simulink model "franka_placement_task"  (R2020b)
settings: Solver=FixedStepAuto  StartTime=0.0  StopTime=20  FixedStep=0.01  RelTol=1e-3
values from neighbouring files (symbols this model uses):
  a0 = 0.99    [init.m]
  berta = 0.98    [init.m]
  csi = 1    [init.m]
  e_max = 0.01    [init.m]
  F_int_max = 5    [init.m]
  F_max = 2    [init.m]
  g = 9.81    [init.m]
  k_can = 500    [init.m]
  k_shelf = k_table    (= 10000)    [init.m]
  k_table = 10000    [init.m]
  k_wall = k_table    (= 10000)    [init.m]
  l_can = 0.1    [init.m]
  M = 1    [init.m]
  mass = 1    [init.m]
  mass_can = 0.5    [init.m]
  q_max = q_max - deg2rad([0 0 0 10 0 5 0])    [init.m]
  q_min = q_min + deg2rad([0 0 0 10 0 5 0])    [init.m]
  y_can = 0.2    [init.m]
  y_wall = -0.3    [init.m]
  z_shelf = 0.3+0.043    (= 0.343)    [init.m]
  z_table = 0+0.043    (= 0.043)    [init.m]
(part 1 of 2)
settings Model: Creator=Rachele  LastModifiedBy=giorg

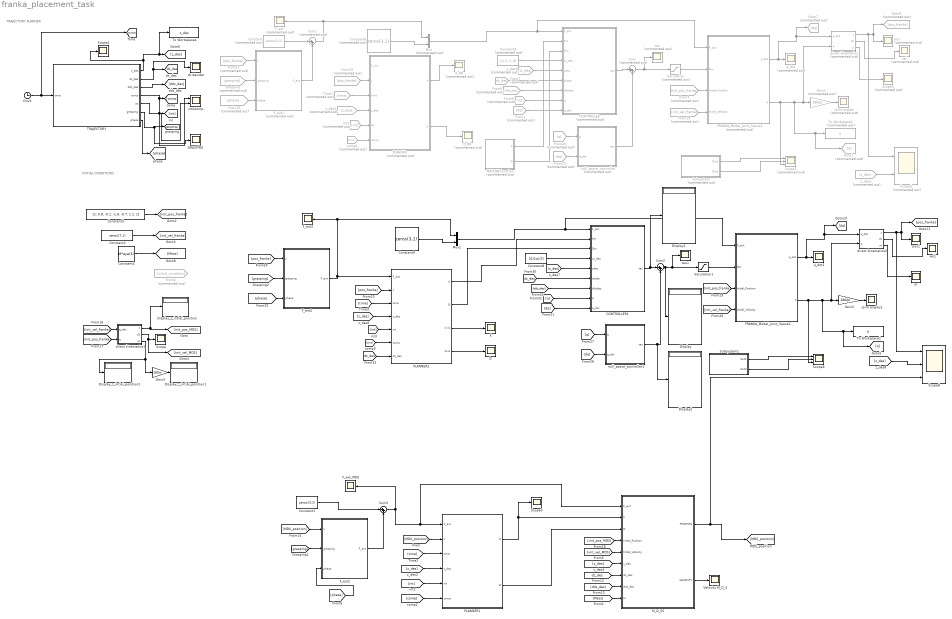
== system franka_placement_task ==
  note: TRAJECTORY PLANNER
  note: INITIAL CONDITIONS
  CONTROLLER : MATLAB Function  Commented=on  TreatAsAtomicUnit=on
  CONTROLLER1 : MATLAB Function  TreatAsAtomicUnit=on
  Clock : Clock
  Constant : Constant  Commented=on  Value=zeros(3,1)
  Constant1 : Constant  Value=zeros(3,1)
  Constant2 : Constant  Value=zeros(7,1)
  Constant3 : Constant  Value=[1; 0.8; -0.1; -1.6; -0.7; 1.1; 1]  VectorParams1D=off
  Constant4 : Constant  Value=M*eye(3)
  Constant5 : Constant  Commented=on  Value=[-2.3; 1; 0]
  Constant6 : Constant  Commented=on  Value=zeros(3,1)
  Constant8 : Constant  Value=[0;0;pi/2]
  Constant9 : Constant  Value=zeros(3,1)
  D : Scope
  D_RR : Scope  Commented=on
  Display : Display
  Display1 : Display
  Display2 : Display
  Display_z_intial_position : Display
  Display_z_intial_position1 : Display
  Display_z_intial_position2 : Display
  FRANKA_Model_Joint_Space1 : Subsystem  Commented=on
  FRANKA_Model_Joint_Space2 : Subsystem
  F_ext : Scope  Commented=on
  F_ext1 : MATLAB Function  Commented=on  TreatAsAtomicUnit=on
  F_ext2 : MATLAB Function  TreatAsAtomicUnit=on
  F_ext3 : Scope
  F_ext4 : MATLAB Function  TreatAsAtomicUnit=on
  F_ext_MDS : Scope
  From1 : From  Commented=on  GotoTag=dq
  From10 : From  Commented=on  GotoTag=pos_franka
  From11 : From  Commented=on  GotoTag=pos_franka
  From15 : From  Commented=on  GotoTag=phase
  From19 : From  Commented=on  GotoTag=init_vel_franka
  From20 : From  Commented=on  GotoTag=q
  From22 : From  Commented=on  GotoTag=dq
  From3 : From  Commented=on  GotoTag=init_pos_franka
  From4 : From  Commented=on  GotoTag=initial_condition
  From7 : From  Commented=on  GotoTag=dz_des  TagVisibility=global
  From8 : From  Commented=on  GotoTag=ddz_des
  From9 : From  Commented=on  GotoTag=q
  GRASPING : Scope
  Gain1 : Gain  Commented=on  Gain=180/pi
  Gain2 : Gain  Gain=180/pi
  Gain3 : Gain  Gain=180/pi
  Goto1 : Goto  Commented=on  GotoTag=q
  Goto7 : Goto  Commented=on  GotoTag=dq
  Goto9 : Goto  Commented=on  GotoTag=pos_franka
  Grasping : From  Commented=on  GotoTag=grasping
  Joint angles : Scope  Commented=on
  Joint angles1 : Scope
  K : Scope
  K_RR : Scope  Commented=on
  MATLAB Function : MATLAB Function  Commented=on  TreatAsAtomicUnit=on
  M_D_S5 : Subsystem
  Mux : Mux  Commented=on  Inputs=2
  Mux1 : Mux  Inputs=2
  PLANNER : Subsystem  Commented=on
  PLANNER1 : Subsystem
  PLANNER2 : Subsystem
  Saturation : Saturate  Commented=on  UpperLimit=100  LowerLimit=-100
  Saturation1 : Saturate  UpperLimit=100  LowerLimit=-100
  Scope : Scope
  Scope1 : Scope  Commented=on  NumInputPorts=3
  Scope2 : Scope  Commented=on
  Scope3 : Scope
  Scope4 : Scope
  Scope5 : Scope  Commented=on  NumInputPorts=2
  Scope6 : Scope  NumInputPorts=3
  Scope8 : Scope  NumInputPorts=3
  Subsystem : Subsystem  Commented=on
  Subsystem1 : Subsystem
  Sum : Sum  Commented=on  Inputs=|++
  Sum1 : Sum  Commented=on  Inputs=|++
  Sum2 : Sum  Inputs=|++
  Sum3 : Sum  Inputs=|++
  TRAJECTORY : Subsystem
  Time1 : From  Commented=on  GotoTag=time
  To Workspace1 : ToWorkspace  VariableName=q  SaveFormat=Timeseries  SampleTime=-1
  To Workspace2 : ToWorkspace  Commented=on  VariableName=q  SaveFormat=Timeseries  SampleTime=-1
  To Workspace4 : ToWorkspace  VariableName=z_des  SaveFormat=Timeseries  SampleTime=-1
      settings: Save2DSignal=2-D array (concatenate along first dimension)
  Velocity M_D_S : Scope
  comp1 : From  Commented=on  GotoTag=comp
  direct kinematics : MATLAB Function  Commented=on  TreatAsAtomicUnit=on
  direct kinematics1 : MATLAB Function  TreatAsAtomicUnit=on
  direct kinematics2 : MATLAB Function  TreatAsAtomicUnit=on
  dz desider : Scope
  int&comp : Scope  NumInputPorts=2
  int1 : From  Commented=on  GotoTag=int
  null_space_controller : MATLAB Function  Commented=on  TreatAsAtomicUnit=on
  null_space_controller1 : MATLAB Function  TreatAsAtomicUnit=on
  or : Scope
  pos : Scope  Commented=on
  pos1 : Scope
  q_dot : Scope  Commented=on
  q_dot1 : Scope
  tau : Scope  Commented=on
  tau1 : Scope
  vel : Scope  Commented=on
  vel1 : Scope
  z_des1 : From  Commented=on  GotoTag=z_des
  z_des3 : From  Commented=on  GotoTag=z_des
  z_des5 : From  Commented=on  GotoTag=z_des
  tag scope: dz_des=global
  wires:
  TRAJECTORY/1(z_des) -> [z_des], To Workspace4/1, Scope4/1
  Sum3/1 -> F_ext_MDS/1, M_D_S5/1(F_ext), PLANNER1/1(F_ext)
  null_space_controller/1(tau) -> Sum/2
  Sum1/1 -> Mux/1, F_ext/1
  Subsystem/2(Out2) -> Scope1/2
  comp1/1 -> PLANNER/6(comp)
  [int] -> PLANNER1/5(int)
  F_ext2/1(F_ext) -> Sum3/2
  PLANNER/1(K) -> K_RR/1
  F_ext1/1(F_ext) -> Sum1/2
  Subsystem/1(Out1) -> Scope1/1
  PLANNER1/1(K) -> M_D_S5/2(K), Scope3/1
  [init_vel_franka] -> direct kinematics1/1(q_dot)
  From11/1 -> F_ext1/1(z)
  Gain1/1 -> Joint angles/1
  Constant1/1 -> Sum3/1
  Constant3/1 -> [init_pos_franka]
  From8/1 -> CONTROLLER/7(ddzdes)
  [phase] -> F_ext2/3(phase)
  Constant/1 -> Sum1/1
  [MDS_position] -> PLANNER1/2(z)
  Saturation/1 -> FRANKA_Model_Joint_Space1/2(tau)
  Grasping/1 -> F_ext1/2(grasping)
  Clock/1 -> TRAJECTORY/1(time), [time]
  [init_vel_MDS] -> M_D_S5/5(Initial_Velocity)
  From20/1 -> null_space_controller/1(q)
  CONTROLLER/1(tau) -> Sum/1
  PLANNER/2(D) -> D_RR/1
  z_des3/1 -> CONTROLLER/5(zdes)
  FRANKA_Model_Joint_Space1/2(q) -> Scope1/3, Goto1/1, To Workspace2/1, direct kinematics/2(q), Gain1/1
  Sum/1 -> Saturation/1, tau/1
  From3/1 -> FRANKA_Model_Joint_Space1/3(Initial_Position)
  direct kinematics1/1(z) -> [init_pos_MDS], Display_z_intial_position/1
  Constant4/1 -> [Mass]
  TRAJECTORY/5(int) -> int&comp/2, [int]
  [init_pos_franka] -> direct kinematics1/2(q)
  direct kinematics/1(z) -> Scope5/1, pos/1, Goto9/1
  From19/1 -> FRANKA_Model_Joint_Space1/4(Initial_Velocity)
  FRANKA_Model_Joint_Space1/1(q_dot) -> Goto7/1, direct kinematics/1(q_dot), q_dot/1
  [dz_des] -> M_D_S5/7(dz_des)
  int1/1 -> PLANNER/5(int)
  [z_des] -> PLANNER1/4(z_des)
  [comp] -> PLANNER1/6(comp)
  [ddz_des] -> M_D_S5/8(ddz_des)
  Time1/1 -> PLANNER/3(time)
  M_D_S5/2(VELOCITY) -> Velocity M_D_S/1
  TRAJECTORY/4(comp) -> int&comp/1, [comp]
  z_des1/1 -> PLANNER/4(z_des)
  From15/1 -> F_ext1/3(phase)
  [time] -> PLANNER1/3(time)
  TRAJECTORY/3(ddz_des) -> [ddz_des]
  [Mass] -> M_D_S5/9(M)
  TRAJECTORY/7(phase) -> [phase]
  [init_pos_MDS] -> M_D_S5/4(Initial_Position)
  TRAJECTORY/2(dz_des) -> dz desider/1, [dz_des]
  direct kinematics/2(dz) -> vel/1
  [MDS_position] -> F_ext2/1(z)
  Constant2/1 -> [init_vel_franka]
  From10/1 -> PLANNER/2(z)
  From9/1 -> CONTROLLER/8(q)
  [z_des] -> M_D_S5/6(z_des)
  TRAJECTORY/6(grasping) -> GRASPING/1, [grasping]
  M_D_S5/1(POSITION) -> Scope8/3, [MDS_position]
  From7/1 -> CONTROLLER/6(dzdes)
  From1/1 -> CONTROLLER/9(q_dot)
  From22/1 -> null_space_controller/2(q_dot)
  [grasping] -> F_ext2/2(grasping)
  Constant5/1 -> CONTROLLER/4(or_des)
  MATLAB Function/1(K) -> CONTROLLER/2(Km)
  MATLAB Function/2(D) -> CONTROLLER/3(Dm)
  direct kinematics/3(or) -> Scope2/1
  z_des5/1 -> Scope5/2
  Constant6/1 -> Mux/2
  Mux/1 -> FRANKA_Model_Joint_Space1/1(F_ext), CONTROLLER/1(F_ext)
  [comp] -> PLANNER2/6(comp)
  Subsystem1/1(Out1) -> Scope6/1
  Mux1/1 -> FRANKA_Model_Joint_Space2/1(F_ext), CONTROLLER1/1(F_ext)
  Constant9/1 -> Mux1/2
  direct kinematics2/3(or) -> or/1
  Constant8/1 -> CONTROLLER1/4(or_des)
  [dq] -> CONTROLLER1/9(q_dot)
  direct kinematics2/2(dz) -> vel1/1
  [ddz_des] -> CONTROLLER1/7(ddzdes)
  [z_des] -> PLANNER2/4(z_des)
  Gain2/1 -> Joint angles1/1
  [dq] -> null_space_controller1/2(q_dot)
  [pos_franka] -> F_ext4/1(z)
  [phase] -> F_ext4/3(phase)
  [time] -> PLANNER2/3(time)
  [pos_franka] -> PLANNER2/2(z)
  [init_pos_franka] -> FRANKA_Model_Joint_Space2/3(Initial_Position)
  FRANKA_Model_Joint_Space2/1(q_dot) -> [dq], direct kinematics2/1(q_dot), q_dot1/1
  direct kinematics2/1(z) -> Scope8/1, pos1/1, [pos_franka]
  [int] -> PLANNER2/5(int)
  [z_des] -> Scope8/2
  [z_des] -> CONTROLLER1/5(zdes)
  null_space_controller1/1(tau) -> Display2/1, Sum2/2
  [grasping] -> F_ext4/2(grasping)
  Sum2/1 -> Display/1, Saturation1/1, tau1/1
  PLANNER2/1(K) -> CONTROLLER1/2(Km)
  FRANKA_Model_Joint_Space2/2(q) -> Scope6/3, [q], To Workspace1/1, direct kinematics2/2(q), Gain2/1
  [dz_des] -> CONTROLLER1/6(dzdes)
  [q] -> null_space_controller1/1(q)
  PLANNER2/2(D) -> CONTROLLER1/3(Dm)
  [init_vel_franka] -> FRANKA_Model_Joint_Space2/4(Initial_Velocity)
  CONTROLLER1/1(tau) -> Display1/1, Sum2/1
  Saturation1/1 -> FRANKA_Model_Joint_Space2/2(tau)
  Subsystem1/2(Out2) -> Scope6/2
  [q] -> CONTROLLER1/8(q)
  PLANNER1/2(D) -> M_D_S5/3(D)
  direct kinematics1/2(dz) -> Scope/1, [init_vel_MDS]
  Gain3/1 -> Display_z_intial_position1/1
  direct kinematics1/3(or) -> Display_z_intial_position2/1, Gain3/1
  F_ext4/1(F_ext) -> PLANNER2/1(F_ext), F_ext3/1, Mux1/1
  PLANNER2/3(kvis) -> K/1
  PLANNER2/4(dvis) -> D/1
  [dz_des] -> PLANNER2/7(dz_des)

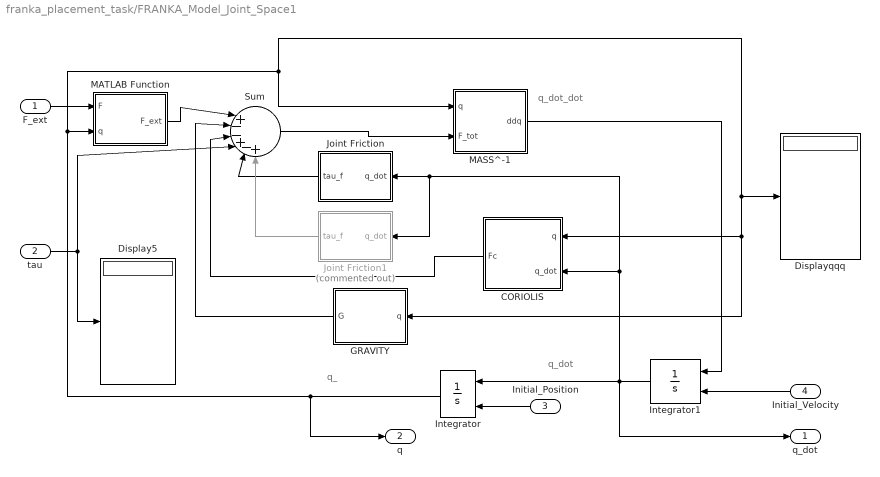
== system franka_placement_task/FRANKA_Model_Joint_Space1 ==
  note: q_dot
  note: q_dot_dot
  note: q_
  F_ext : Inport
  tau : Inport  Port=2
  Initial_Position : Inport  Port=3
  Initial_Velocity : Inport  Port=4
  CORIOLIS : MATLAB Function  TreatAsAtomicUnit=on
  Display5 : Display
  Displayqqq : Display
  GRAVITY : MATLAB Function  TreatAsAtomicUnit=on
  Integrator : Integrator  InitialConditionSource=external
  Integrator1 : Integrator  InitialConditionSource=external  InitialCondition=[0;0]
  Joint Friction : MATLAB Function  TreatAsAtomicUnit=on
  Joint Friction1 : MATLAB Function  Commented=on  TreatAsAtomicUnit=on
  MASS^-1 : MATLAB Function  TreatAsAtomicUnit=on
  MATLAB Function : MATLAB Function  TreatAsAtomicUnit=on
  Sum : Sum  Inputs=||+--+-+
  q_dot : Outport
  q : Outport  Port=2
  wires:
  GRAVITY/1(G) -> Sum/2
  MATLAB Function/1(F_ext) -> Sum/1
  Initial_Position/1 -> Integrator/2
  F_ext/1 -> MATLAB Function/1(F)
  Integrator/1 -> MASS^-1/1(q), GRAVITY/1(q), CORIOLIS/1(q), Displayqqq/1, MATLAB Function/2(q), q/1
  Integrator1/1 -> q_dot/1, CORIOLIS/2(q_dot), Joint Friction1/1(q_dot), Joint Friction/1(q_dot), Integrator/1
  Initial_Velocity/1 -> Integrator1/2
  MASS^-1/1(ddq) -> Integrator1/1
  Sum/1 -> MASS^-1/2(F_tot)
  CORIOLIS/1(Fc) -> Sum/3
  tau/1 -> Display5/1, Sum/4
  Joint Friction/1(tau_f) -> Sum/5
  Joint Friction1/1(tau_f) -> Sum/6

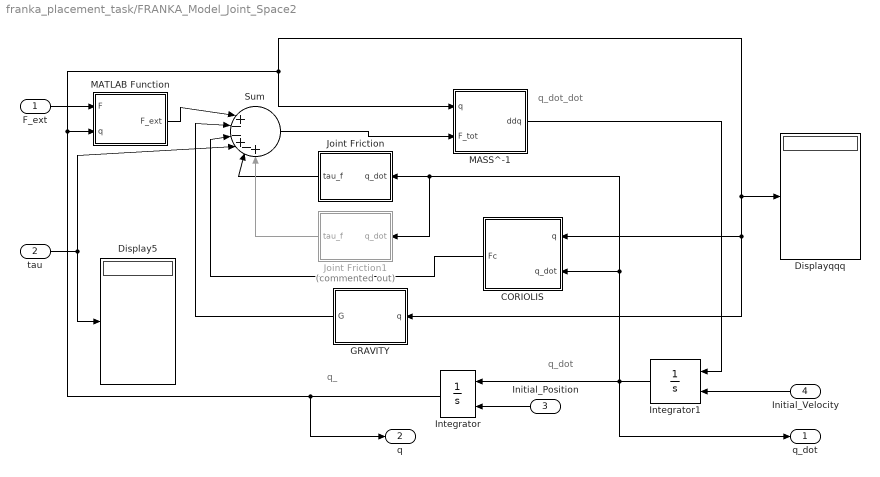
== system franka_placement_task/FRANKA_Model_Joint_Space2 ==
  note: q_dot
  note: q_dot_dot
  note: q_
  F_ext : Inport
  tau : Inport  Port=2
  Initial_Position : Inport  Port=3
  Initial_Velocity : Inport  Port=4
  CORIOLIS : MATLAB Function  TreatAsAtomicUnit=on
  Display5 : Display
  Displayqqq : Display
  GRAVITY : MATLAB Function  TreatAsAtomicUnit=on
  Integrator : Integrator  InitialConditionSource=external
  Integrator1 : Integrator  InitialConditionSource=external  InitialCondition=[0;0]
  Joint Friction : MATLAB Function  TreatAsAtomicUnit=on
  Joint Friction1 : MATLAB Function  Commented=on  TreatAsAtomicUnit=on
  MASS^-1 : MATLAB Function  TreatAsAtomicUnit=on
  MATLAB Function : MATLAB Function  TreatAsAtomicUnit=on
  Sum : Sum  Inputs=||+--+-+
  q_dot : Outport
  q : Outport  Port=2
  wires:
  GRAVITY/1(G) -> Sum/2
  MATLAB Function/1(F_ext) -> Sum/1
  Initial_Position/1 -> Integrator/2
  F_ext/1 -> MATLAB Function/1(F)
  Integrator/1 -> MASS^-1/1(q), GRAVITY/1(q), CORIOLIS/1(q), Displayqqq/1, MATLAB Function/2(q), q/1
  Integrator1/1 -> q_dot/1, CORIOLIS/2(q_dot), Joint Friction1/1(q_dot), Joint Friction/1(q_dot), Integrator/1
  Initial_Velocity/1 -> Integrator1/2
  MASS^-1/1(ddq) -> Integrator1/1
  Sum/1 -> MASS^-1/2(F_tot)
  CORIOLIS/1(Fc) -> Sum/3
  tau/1 -> Display5/1, Sum/4
  Joint Friction/1(tau_f) -> Sum/5
  Joint Friction1/1(tau_f) -> Sum/6

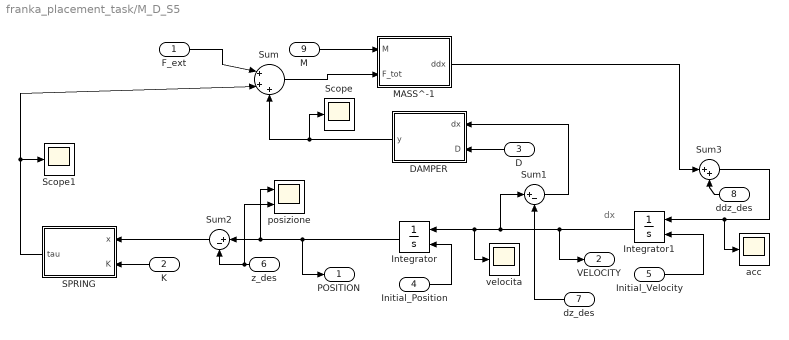
== system franka_placement_task/M_D_S5 ==
  note: dx
  F_ext : Inport
  K : Inport  Port=2
  D : Inport  Port=3
  Initial_Position : Inport  Port=4
  Initial_Velocity : Inport  Port=5
  z_des : Inport  Port=6
  dz_des : Inport  Port=7
  ddz_des : Inport  Port=8
  M : Inport  Port=9
  DAMPER : MATLAB Function  TreatAsAtomicUnit=on
  Integrator : Integrator  InitialConditionSource=external
  Integrator1 : Integrator  InitialConditionSource=external
  MASS^-1 : MATLAB Function  TreatAsAtomicUnit=on
  SPRING : MATLAB Function  TreatAsAtomicUnit=on
  Scope : Scope
  Scope1 : Scope
  Sum : Sum  Inputs=|+++
  Sum1 : Sum  Inputs=|+-
  Sum2 : Sum  Inputs=|+-
  Sum3 : Sum  Inputs=|++
  acc : Scope
  posizione : Scope  NumInputPorts=2
  velocita : Scope
  POSITION : Outport
  VELOCITY : Outport  Port=2
  wires:
  Integrator1/1 -> velocita/1, Integrator/1, Sum1/1, VELOCITY/1
  SPRING/1(tau) -> Sum/2, Scope1/1
  Integrator/1 -> posizione/1, Sum2/1, POSITION/1
  DAMPER/1(y) -> Scope/1, Sum/3
  Sum/1 -> MASS^-1/2(F_tot)
  M/1 -> MASS^-1/1(M)
  D/1 -> DAMPER/2(D)
  K/1 -> SPRING/2(K)
  Initial_Velocity/1 -> Integrator1/2
  Initial_Position/1 -> Integrator/2
  z_des/1 -> posizione/2, Sum2/2
  Sum2/1 -> SPRING/1(x)
  MASS^-1/1(ddx) -> Sum3/1
  Sum1/1 -> DAMPER/1(dx)
  Sum3/1 -> acc/1, Integrator1/1
  dz_des/1 -> Sum1/2
  ddz_des/1 -> Sum3/2
  F_ext/1 -> Sum/1

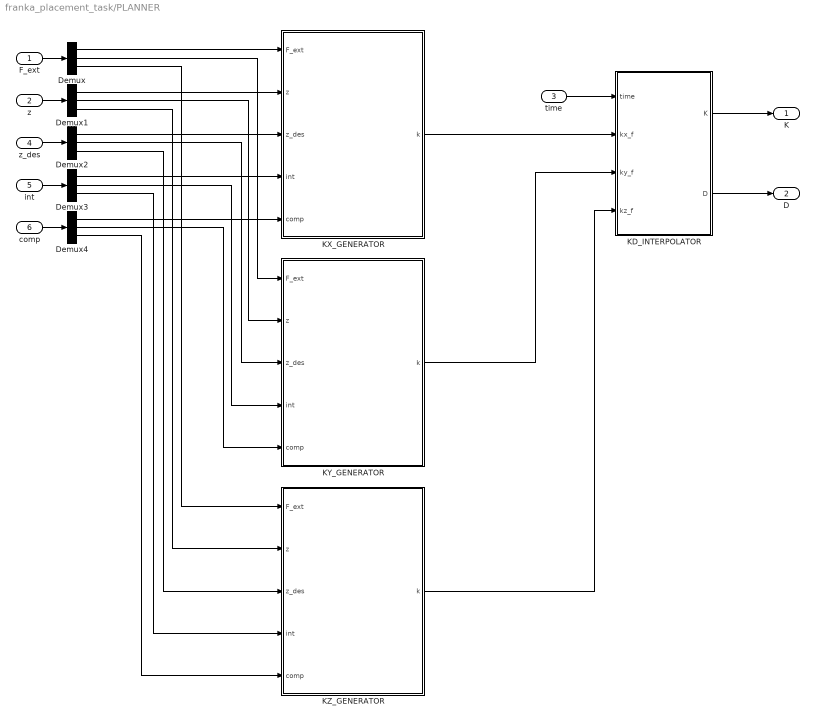
== system franka_placement_task/PLANNER ==
  F_ext : Inport
  z : Inport  Port=2
  time : Inport  Port=3
  z_des : Inport  Port=4
  int : Inport  Port=5
  comp : Inport  Port=6
  Demux{,1..4} (5 alike) : Demux  Outputs=3
  "KD_INTERPOLATOR " : MATLAB Function  TreatAsAtomicUnit=on
  KX_GENERATOR : MATLAB Function  TreatAsAtomicUnit=on
  KY_GENERATOR : MATLAB Function  TreatAsAtomicUnit=on
  KZ_GENERATOR : MATLAB Function  TreatAsAtomicUnit=on
  K : Outport
  D : Outport  Port=2
  wires:
  time/1 -> "KD_INTERPOLATOR "/1(time)
  "KD_INTERPOLATOR "/2(D) -> D/1
  "KD_INTERPOLATOR "/1(K) -> K/1
  KX_GENERATOR/1(k) -> "KD_INTERPOLATOR "/2(kx_f)
  Demux/1 -> KX_GENERATOR/1(F_ext)
  Demux1/1 -> KX_GENERATOR/2(z)
  Demux2/1 -> KX_GENERATOR/3(z_des)
  Demux3/1 -> KX_GENERATOR/4(int)
  Demux4/1 -> KX_GENERATOR/5(comp)
  F_ext/1 -> Demux/1
  z/1 -> Demux1/1
  z_des/1 -> Demux2/1
  int/1 -> Demux3/1
  comp/1 -> Demux4/1
  Demux/2 -> KY_GENERATOR/1(F_ext)
  Demux1/2 -> KY_GENERATOR/2(z)
  Demux2/2 -> KY_GENERATOR/3(z_des)
  Demux3/2 -> KY_GENERATOR/4(int)
  Demux4/2 -> KY_GENERATOR/5(comp)
  Demux/3 -> KZ_GENERATOR/1(F_ext)
  Demux1/3 -> KZ_GENERATOR/2(z)
  Demux2/3 -> KZ_GENERATOR/3(z_des)
  Demux3/3 -> KZ_GENERATOR/4(int)
  Demux4/3 -> KZ_GENERATOR/5(comp)
  KY_GENERATOR/1(k) -> "KD_INTERPOLATOR "/3(ky_f)
  KZ_GENERATOR/1(k) -> "KD_INTERPOLATOR "/4(kz_f)

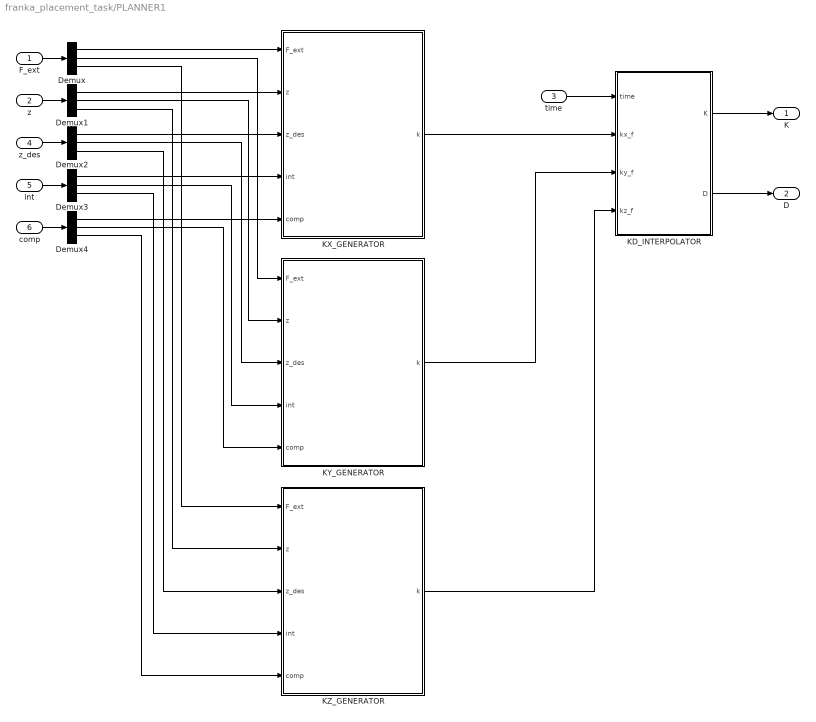
== system franka_placement_task/PLANNER1 ==
  F_ext : Inport
  z : Inport  Port=2
  time : Inport  Port=3
  z_des : Inport  Port=4
  int : Inport  Port=5
  comp : Inport  Port=6
  Demux{,1..4} (5 alike) : Demux  Outputs=3
  "KD_INTERPOLATOR " : MATLAB Function  TreatAsAtomicUnit=on
  KX_GENERATOR : MATLAB Function  TreatAsAtomicUnit=on
  KY_GENERATOR : MATLAB Function  TreatAsAtomicUnit=on
  KZ_GENERATOR : MATLAB Function  TreatAsAtomicUnit=on
  K : Outport
  D : Outport  Port=2
  wires:
  KZ_GENERATOR/1(k) -> "KD_INTERPOLATOR "/4(kz_f)
  KY_GENERATOR/1(k) -> "KD_INTERPOLATOR "/3(ky_f)
  Demux4/3 -> KZ_GENERATOR/5(comp)
  Demux3/3 -> KZ_GENERATOR/4(int)
  Demux2/3 -> KZ_GENERATOR/3(z_des)
  Demux1/3 -> KZ_GENERATOR/2(z)
  Demux/3 -> KZ_GENERATOR/1(F_ext)
  Demux4/2 -> KY_GENERATOR/5(comp)
  Demux3/2 -> KY_GENERATOR/4(int)
  Demux2/2 -> KY_GENERATOR/3(z_des)
  Demux1/2 -> KY_GENERATOR/2(z)
  Demux/2 -> KY_GENERATOR/1(F_ext)
  comp/1 -> Demux4/1
  int/1 -> Demux3/1
  z_des/1 -> Demux2/1
  z/1 -> Demux1/1
  F_ext/1 -> Demux/1
  Demux4/1 -> KX_GENERATOR/5(comp)
  Demux3/1 -> KX_GENERATOR/4(int)
  Demux2/1 -> KX_GENERATOR/3(z_des)
  Demux1/1 -> KX_GENERATOR/2(z)
  Demux/1 -> KX_GENERATOR/1(F_ext)
  KX_GENERATOR/1(k) -> "KD_INTERPOLATOR "/2(kx_f)
  "KD_INTERPOLATOR "/1(K) -> K/1
  "KD_INTERPOLATOR "/2(D) -> D/1
  time/1 -> "KD_INTERPOLATOR "/1(time)

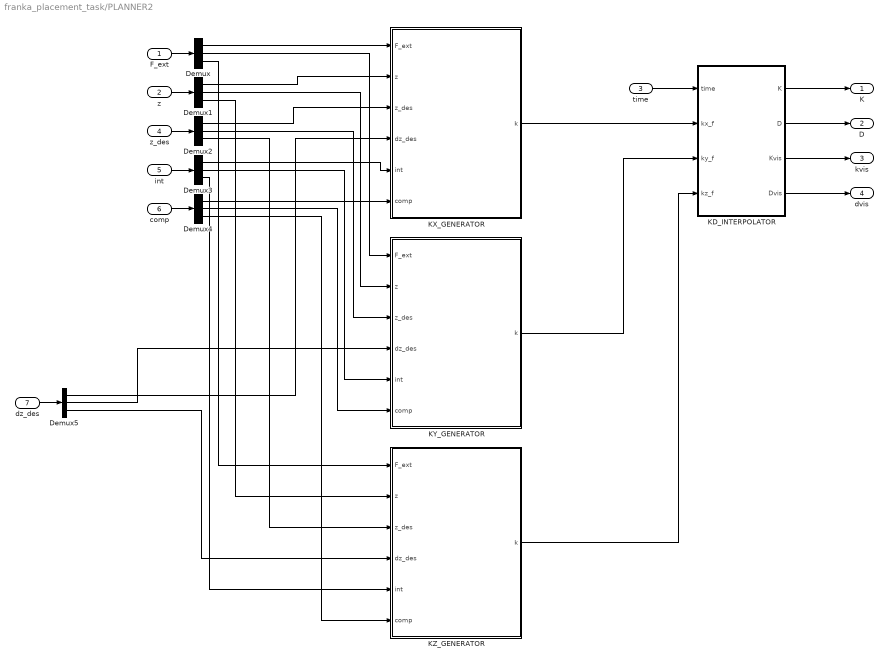
== system franka_placement_task/PLANNER2 ==
  F_ext : Inport
  z : Inport  Port=2
  time : Inport  Port=3
  z_des : Inport  Port=4
  int : Inport  Port=5
  comp : Inport  Port=6
  dz_des : Inport  Port=7
  Demux{,1..5} (6 alike) : Demux  Outputs=3
  "KD_INTERPOLATOR " : MATLAB Function  TreatAsAtomicUnit=on
  KX_GENERATOR : MATLAB Function  TreatAsAtomicUnit=on
  KY_GENERATOR : MATLAB Function  TreatAsAtomicUnit=on
  KZ_GENERATOR : MATLAB Function  TreatAsAtomicUnit=on
  K : Outport
  D : Outport  Port=2
  kvis : Outport  Port=3
  dvis : Outport  Port=4
  wires:
  time/1 -> "KD_INTERPOLATOR "/1(time)
  "KD_INTERPOLATOR "/2(D) -> D/1
  "KD_INTERPOLATOR "/1(K) -> K/1
  KX_GENERATOR/1(k) -> "KD_INTERPOLATOR "/2(kx_f)
  Demux/1 -> KX_GENERATOR/1(F_ext)
  Demux1/1 -> KX_GENERATOR/2(z)
  Demux2/1 -> KX_GENERATOR/3(z_des)
  Demux3/1 -> KX_GENERATOR/5(int)
  Demux4/1 -> KX_GENERATOR/6(comp)
  F_ext/1 -> Demux/1
  z/1 -> Demux1/1
  z_des/1 -> Demux2/1
  int/1 -> Demux3/1
  comp/1 -> Demux4/1
  Demux/2 -> KY_GENERATOR/1(F_ext)
  Demux1/2 -> KY_GENERATOR/2(z)
  Demux2/2 -> KY_GENERATOR/3(z_des)
  Demux3/2 -> KY_GENERATOR/5(int)
  Demux4/2 -> KY_GENERATOR/6(comp)
  Demux/3 -> KZ_GENERATOR/1(F_ext)
  Demux1/3 -> KZ_GENERATOR/2(z)
  Demux2/3 -> KZ_GENERATOR/3(z_des)
  Demux3/3 -> KZ_GENERATOR/5(int)
  Demux4/3 -> KZ_GENERATOR/6(comp)
  KY_GENERATOR/1(k) -> "KD_INTERPOLATOR "/3(ky_f)
  KZ_GENERATOR/1(k) -> "KD_INTERPOLATOR "/4(kz_f)
  "KD_INTERPOLATOR "/3(Kvis) -> kvis/1
  "KD_INTERPOLATOR "/4(Dvis) -> dvis/1
  dz_des/1 -> Demux5/1
  Demux5/3 -> KZ_GENERATOR/4(dz_des)
  Demux5/1 -> KX_GENERATOR/4(dz_des)
  Demux5/2 -> KY_GENERATOR/4(dz_des)

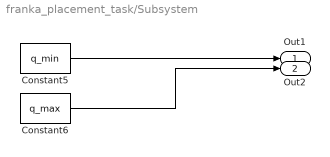
== system franka_placement_task/Subsystem ==
  Constant5 : Constant  Value=q_min
  Constant6 : Constant  Value=q_max
  Out1 : Outport
  Out2 : Outport  Port=2
  wires:
  Constant5/1 -> Out1/1
  Constant6/1 -> Out2/1

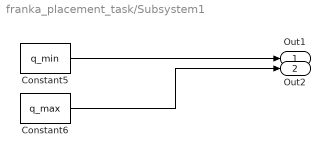
== system franka_placement_task/Subsystem1 ==
  Constant5 : Constant  Value=q_min
  Constant6 : Constant  Value=q_max
  Out1 : Outport
  Out2 : Outport  Port=2
  wires:
  Constant5/1 -> Out1/1
  Constant6/1 -> Out2/1

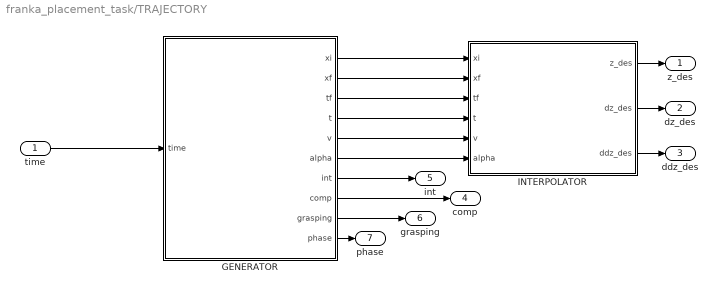
== system franka_placement_task/TRAJECTORY ==
  time : Inport
  GENERATOR : MATLAB Function  TreatAsAtomicUnit=on
  INTERPOLATOR : MATLAB Function  TreatAsAtomicUnit=on
  z_des : Outport
  dz_des : Outport  Port=2
  ddz_des : Outport  Port=3
  comp : Outport  Port=4
  int : Outport  Port=5
  grasping : Outport  Port=6
  phase : Outport  Port=7
  wires:
  GENERATOR/1(xi) -> INTERPOLATOR/1(xi)
  GENERATOR/2(xf) -> INTERPOLATOR/2(xf)
  GENERATOR/3(tf) -> INTERPOLATOR/3(tf)
  GENERATOR/4(t) -> INTERPOLATOR/4(t)
  GENERATOR/5(v) -> INTERPOLATOR/5(v)
  GENERATOR/6(alpha) -> INTERPOLATOR/6(alpha)
  INTERPOLATOR/1(z_des) -> z_des/1
  INTERPOLATOR/2(dz_des) -> dz_des/1
  INTERPOLATOR/3(ddz_des) -> ddz_des/1
  GENERATOR/7(int) -> int/1
  GENERATOR/8(comp) -> comp/1
  GENERATOR/9(grasping) -> grasping/1
  GENERATOR/10(phase) -> phase/1
  time/1 -> GENERATOR/1(time)

== matlab function franka_placement_task/PLANNER1/KD_INTERPOLATOR  ==
  settings: updateMethod=DISCRETE  sampleTime=Ts
  data: time input; K output; kx_f input; ky_f input; kz_f input; D output; e_max parameter; F_max parameter; M parameter; berta parameter; a0 parameter; mass parameter; csi parameter
function [K,D] = fcn(time, kx_f, ky_f, kz_f, e_max, F_max, M, berta, a0, mass, csi)
%% Description
% Interpolate K in order to guarantee stability

%% Outputs
% K             Stiffness matrix
% D             Damping matrix

%% Inputs
% kx_f, ky, f   desired values of K

%% Parameters
% F_max         nominal disturbance forces
% e_max         maximum steady-state error
% M             virtual mass
% berta, a0     parameters for the computation of stability conditions
% mass          virtual mass

%% persistent initialization
persistent kx ky kz time_prec
if isempty(time_prec)
    time_prec = 0;              % previous simulation time
end
if isempty(kx)
   kx = F_max/e_max;         % last value of k
end
if isempty(ky)
   ky = F_max/e_max;
end
if isempty(kz)
   kz = F_max/e_max;
end

% set k from desired one 
if kx_f <= kx       
    kx = kx_f;
else 
    % increese k in accordance with the stability conditions
    kx_i = kx;
    k_dotx = berta*(4*a0*sqrt(kx_i/mass)*(kx_i)^(3/2))/(sqrt(kx_i) + 2*a0*csi*sqrt(kx_i));
    k_tempx = kx_i + k_dotx*(time -time_prec);
    if k_tempx > kx_f
        kx = kx_f;
    else
        kx = k_tempx;
    end
end

% Y axes, same as X axes
if ky_f <= ky
    ky = ky_f;
else 
    ky_i = ky;
    k_doty = berta*(4*a0*sqrt(ky_i/mass)*(ky_i)^(3/2))/(sqrt(ky_i) + 2*a0*csi*sqrt(ky_i));
    k_tempy = ky_i + k_doty*(time -time_prec);
    if k_tempy > ky_f
        ky = ky_f;
    else
        ky = k_tempy;
    end
end

% Z axes, same as other axes
if kz_f <= kz
    kz = kz_f;
else 
    kz_i = kz;
    k_dotz = berta*(4*a0*sqrt(kz_i/mass)*(kz_i)^(3/2))/(sqrt(kz_i) + 2*a0*csi*sqrt(kz_i));
    k_tempz = kz_i + k_dotz*(time -time_prec);
    if k_tempz > kz_f
        kz = kz_f;
    else
        kz = k_tempz;
    end
end

time_prec = time;

% damping computation, critically damped condition
dx = sqrt(4*kx*M);
dy = sqrt(4*ky*M);
dz = sqrt(4*kz*M);

%% Final impedance matrices
D = diag([dx, dy, dz]);
K = diag([kx, ky, kz]);

end

== matlab function franka_placement_task/PLANNER1/KX_GENERATOR ==
  settings: updateMethod=DISCRETE  sampleTime=Ts
  data: k output; F_ext input; z input; z_des input; int input; comp input; e_max parameter; F_max parameter; F_int_max parameter
function k = fcn(F_ext, z, z_des, int, comp, e_max, F_max, F_int_max)
%% Description
% Set the K coefficient for a variable impedance controller based on a
% desired trajectory

%% Outputs
% k             stiffness

%% Inputs
% F_ext         measured external force
% z_des         desired trajectory
% z             current position
% int, comp     booleans for the interaction and compensation phase

%% Parameters
% F_int_max     desired interaction force
% F_max         nominal disturbance forces
% e_max         maximum steady-state error

%% persistent initialization
persistent ki kc F_comp int_prec comp_prec z_int z_int_dir 
if isempty(ki)
   ki = F_max/e_max;        % k obtained from interaction
end
if isempty(F_comp)
   F_comp = 0;              % weight to compensate
end
if isempty(kc)
      kc = F_max/e_max;     % k obtained from compensation
end
if isempty(z_int) 
    z_int = 1000;       % obstacle(or interaction) position
end
if isempty(z_int_dir) 
    z_int_dir = 0;          % prohibited direction due to the obstacle
end
if isempty(int_prec)
    int_prec = 0;           % previous values of int
end
if isempty(comp_prec)
    comp_prec = 0;          % previous values od comp
end

%% INTERACTION
% set ki in order to match a desired interaction force with the
% envirorment, and store interaction's position when detected
% X axes
if int == 1
    % detection of an interaction 
    if abs(F_ext-F_comp) > F_max
        if z_int == 1000                     % z_int has not been set yet
            z_int = z;
            z_int_dir = -sign(F_ext-F_comp);
        end
    end
    % setting of ki
    if abs(F_ext-F_comp) > F_int_max 
        % if interaction force is higher than threshold
        if ki*abs(z-z_des) > F_int_max
            ktemp_x = F_int_max/abs(z-z_des);
            if ktemp_x < ki                % ki needs to be only decreased
                ki = ktemp_x;
            end
        end
    end
end

%% COMPENSATION
% set kc in order to compensate the effect of the weight of the object,
% and store it
% X axes
if comp == 1
    % compensation detection
    if z_int == 1000                     % z_int not set before
       if abs(F_ext)/kc > e_max         
            kc = abs(F_ext)/e_max;
            F_comp = F_ext;
       end
    else 
        if z_int_dir == 1                % obstacle in above
            if z < z_int
                if abs(F_ext)/kc > e_max 
                    kc = abs(F_ext)/e_max;
                    F_comp = F_ext;
                end
            end
        else                                % obstacle is below
            if z > z_int
                if abs(F_ext)/kc > e_max
                    kc = abs(F_ext)/e_max;
                    F_comp = F_ext;
                end
            end
        end 
   end
end

%% reset to default values when comp or int shifts to zero
if comp==0 && comp_prec==1
    kc = F_max/e_max;
    F_comp = 0;
end
if int==0 && int_prec==1
    ki = F_max/e_max;
end

%% from int to comp and vice versa
if int==1 && int_prec==0
    if comp_prec == 1
        ki = kc;
    end
    z_int=1000;
    z_int_dir=0;
end
if comp == 1 && comp_prec==0
    if int_prec == 1
        kc = ki;
    end
end

% update to last booleans
int_prec = int;
comp_prec = comp;


%% Selection of Final Values of D-K
% default values
k = abs(F_max)/e_max;

% compensation
if comp == 1
    k = kc;
end

% both compensation and interaction are activated
% if "away" from obstacle set k = kc else ki
if int == 1
    k = ki;
    if comp == 1
        if z_int == 1000
            k = kc;                       % obstacle not reached
        else
            if z_int_dir == 1
                if z_des < z_int
                    k = kc;               % obstacle reached but "going away"
                end
            else
                if z_des > z_int
                    k = kc;               % obstacle reached but "going away"
                end
            end
        end
    else
        if z_int == 1000
            k = F_max/e_max;            % restore to default
        else
            if z_int_dir == 1
                if z_des < z_int
                    k = F_max/e_max;    % restore because "going away"
                end
            else
                if z_des > z_int
                    k = F_max/e_max;    % restore because "going away"
                end
            end
        end
    end
end

end

== matlab function franka_placement_task/null_space_controller ==
  data: q input; tau output; q_dot input
function tau = nsc(q, q_dot)
coder.extrinsic('get_Jacobianoa','get_MassMatrix');
Ja = zeros(6,7);
B = zeros(7,7);
q_min = [-2.8973   -1.7628   -2.8973   -3.0718   -2.8973   -0.0175  -2.8973];
q_min = q_min + deg2rad([0 0 0 10 0 5 0]);
%        166.0031  101.0010  166.0031 -3.9992   166.0031   215.0024  166.0031
q_max = [ 2.8973    1.7628    2.8973  -0.0698    2.8973    3.7525    2.8973];
q_max = q_max - deg2rad([0 0 0 10 0 5 0]);

q_des = (q_max + q_min)'/2;

Ja = get_Jacobianoa(q);
B = get_MassMatrix(q);
%Ja_inv = inv(B)*(Ja')*inv(Ja*inv(B)*Ja');
Ja_t_inv = inv(Ja*inv(B)*Ja')*Ja*inv(B); %inertia-weighted pseudo inverse Ja'
Ja_inv = Ja_t_inv'; 
% add joint friction
D_joints = eye(7)*2;
K_joints = eye(7)*10;
%N = eye(7) - Ja_inv*Ja;
N = eye(7) - Ja'*(Ja_t_inv);
tau = N*(K_joints*(q_des - q) -D_joints*q_dot);

end

== matlab function franka_placement_task/FRANKA_Model_Joint_Space1/CORIOLIS ==
  data: q input; Fc output double; q_dot input
function Fc = fcn(q,q_dot)

C = zeros(7,7);

C = get_CoriolisMatrix(q,q_dot);

Fc = C*q_dot;

end

== matlab function franka_placement_task/PLANNER1/KY_GENERATOR ==
  settings: updateMethod=DISCRETE  sampleTime=Ts
  data: k output; F_ext input; z input; z_des input; int input; comp input; e_max parameter; F_max parameter; F_int_max parameter
function k = fcn(F_ext, z, z_des, int, comp, e_max, F_max, F_int_max)
%% Description
% Set the K coefficient for a variable impedance controller based on a
% desired trajectory

%% Outputs
% k             stiffness

%% Inputs
% F_ext         measured external force
% z_des         desired trajectory
% z             current position
% int, comp     booleans for the interaction and compensation phase

%% Parameters
% F_int_max     desired interaction force
% F_max         nominal disturbance forces
% e_max         maximum steady-state error

%% persistent initialization
persistent ki kc F_comp int_prec comp_prec z_int z_int_dir 
if isempty(ki)
   ki = F_max/e_max;        % k obtained from interaction
end
if isempty(F_comp)
   F_comp = 0;              % weight to compensate
end
if isempty(kc)
      kc = F_max/e_max;     % k obtained from compensation
end
if isempty(z_int) 
    z_int = 1000;       % obstacle(or interaction) position
end
if isempty(z_int_dir) 
    z_int_dir = 0;          % prohibited direction due to the obstacle
end
if isempty(int_prec)
    int_prec = 0;           % previous values of int
end
if isempty(comp_prec)
    comp_prec = 0;          % previous values od comp
end

%% INTERACTION
% set ki in order to match a desired interaction force with the
% envirorment, and store interaction's position when detected
% X axes
if int == 1
    % detection of an interaction 
    if abs(F_ext-F_comp) > F_max
        if z_int == 1000                     % z_int has not been set yet
            z_int = z;
            z_int_dir = -sign(F_ext-F_comp);
        end
    end
    % setting of ki
    if abs(F_ext-F_comp) > F_int_max 
        % if interaction force is higher than threshold
        if ki*abs(z-z_des) > F_int_max
            ktemp_x = F_int_max/abs(z-z_des);
            if ktemp_x < ki                % ki needs to be only decreased
                ki = ktemp_x;
            end
        end
    end
end

%% COMPENSATION
% set kc in order to compensate the effect of the weight of the object,
% and store it
% X axes
if comp == 1
    % compensation detection
    if z_int == 1000                     % z_int not set before
       if abs(F_ext)/kc > e_max         
            kc = abs(F_ext)/e_max;
            F_comp = F_ext;
       end
    else 
        if z_int_dir == 1                % obstacle in above
            if z < z_int
                if abs(F_ext)/kc > e_max 
                    kc = abs(F_ext)/e_max;
                    F_comp = F_ext;
                end
            end
        else                                % obstacle is below
            if z > z_int
                if abs(F_ext)/kc > e_max
                    kc = abs(F_ext)/e_max;
                    F_comp = F_ext;
                end
            end
        end 
   end
end

%% reset to default values when comp or int shifts to zero
if comp==0 && comp_prec==1
    kc = F_max/e_max;
    F_comp = 0;
end
if int==0 && int_prec==1
    ki = F_max/e_max;
end

%% from int to comp and vice versa
if int==1 && int_prec==0
    if comp_prec == 1
        ki = kc;
    end
    z_int=1000;
    z_int_dir=0;
end
if comp == 1 && comp_prec==0
    if int_prec == 1
        kc = ki;
    end
end

% update to last booleans
int_prec = int;
comp_prec = comp;


%% Selection of Final Values of D-K
% default values
k = abs(F_max)/e_max;

% compensation
if comp == 1
    k = kc;
end

% both compensation and interaction are activated
% if "away" from obstacle set k = kc else ki
if int == 1
    k = ki;
    if comp == 1
        if z_int == 1000
            k = kc;                       % obstacle not reached
        else
            if z_int_dir == 1
                if z_des < z_int
                    k = kc;               % obstacle reached but "going away"
                end
            else
                if z_des > z_int
                    k = kc;               % obstacle reached but "going away"
                end
            end
        end
    else
        if z_int == 1000
            k = F_max/e_max;            % restore to default
        else
            if z_int_dir == 1
                if z_des < z_int
                    k = F_max/e_max;    % restore because "going away"
                end
            else
                if z_des > z_int
                    k = F_max/e_max;    % restore because "going away"
                end
            end
        end
    end
end

end

== matlab function franka_placement_task/TRAJECTORY/GENERATOR ==
  data: time input; xi output; xf output; tf output; t output; v output; alpha output; int output; comp output; grasping output; phase output
function  [xi, xf, tf, t, v, alpha, int, comp, grasping, phase] = fcn(time)

alpha = 0.1;
phase = 1;
int = [1; 1; 1];
comp = [0; 0; 0];
grasping = 0;

if time >= 0 && time < 4
    tf = 4;
    xi = [0.4; 0.4; 0.2];
    xf = [0.4; 0.1; -0.1];
    t = time;
elseif time >= 4 && time < 5
    tf = 1;
    xf = [0.4; 0.1; -0.1];
    xi = xf; 
    t = time - 4;
elseif time >= 5 && time < 9
    tf = 4;
    xf = [0.4; 0.1; 0.5];
    xi = [0.4; 0.1; -0.1];
    t = time - 5;
    grasping = 1; 
    int = [0; 0; 1];
    comp = [0; 0; 1];
    if time > 8
        int = [0; 0; 0];
    end
elseif time >= 9 && time < 13
    tf = 4; 
    xf = [0.4; -0.4; 0.2];
    xi = [0.4; 0.1; 0.5];
    t = time - 9;
    phase = 2; 
    grasping = 1;
    int = [0; 1; 1];
    comp = [0; 0; 1];
elseif time >= 13 && time < 19
    tf = 6;
    xf = [0.4; 0.1; 0.5];
    xi = [0.4; -0.4; 0.2];
    t = time - 13; 
    phase = 3; 
    grasping = 0; 
    int = [0; 1; 1];
    comp = [0; 0; 0];
else 
    tf = 1000;
    xf = [0.4; 0.1; 0.5];
    xi = xf;
    t = time - 10; 
    phase = 3; 
    grasping = 0; 
    int = [0; 0; 0];
    comp =[0; 0; 0];
end
v = [(xf(1) - xi(1))/((1-alpha)*tf); (xf(2) - xi(2))/((1-alpha)*tf); (xf(3) - xi(3))/((1-alpha)*tf)];
































% if time >= 0 && time < 1
%     tf = 1;
%     xi = [0; 0.3];
%     xf = [0.7; -0.1];
%     v = [(xf(1) - xi(1))/((1-alpha)*tf); (xf(2) - xi(2))/((1-alpha)*tf)];
%     t = time;
% elseif time >= 1 && time < 2
%     tf = 1;
%     xf = [0.7; -0.1];
%     xi = xf; 
%     v = [(xf(1) - xi(1))/((1-alpha)*tf); (xf(2) - xi(2))/((1-alpha)*tf)];
%     t = time - 1;
% elseif time >= 2 && time < 2.5
%     tf = 0.5;
%     xf = [0.7; 1];
%     xi = [0.7; -0.1];
%     v = [(xf(1) - xi(1))/((1-alpha)*tf); (xf(2) - xi(2))/((1-alpha)*tf)];
%     t = time - 2;
%     grasping = 1; 
%     int = [0; 1];
%     comp = [0; 1];
%     if time > 2.49
%         int = [0; 0];
%     end
% elseif time >= 2.5 && time < 3.5
%     tf = 1; 
%     xf = [1.6; 0.4];
%     xi = [0.7; 1];
%     v = [(xf(1) - xi(1))/((1-alpha)*tf); (xf(2) - xi(2))/((1-alpha)*tf)];
%     t = time - 2.5;
%     phase = 2; 
%     grasping = 1;
%     int = [1; 1];
%     comp = [0; 1];
% elseif time >= 3.5 && time < 5
%     tf = 1.5;
%     xf = [0.7; 1];
%     xi = [1.6; 0.4];
%     v = [(xf(1) - xi(1))/((1-alpha)*tf); (xf(2) - xi(2))/((1-alpha)*tf)]; 
%     t = time - 3.5; 
%     phase = 3; 
%     grasping = 0; 
%     int = [1; 1];
%     comp = [0; 0];
% else 
%     tf = 1000;
%     xf = [0.7; 1];
%     xi = xf; 
%     v = [(xf(1) - xi(1))/((1-alpha)*tf); (xf(2) - xi(2))/((1-alpha)*tf)]; 
%     t = time - 5; 
%     phase = 3; 
%     grasping = 0; 
%     int = [0; 0];
%     comp =[0; 0];
% end

end

== matlab function franka_placement_task/direct kinematics ==
  data: q_dot input double; q input double; z output double; dz output double; or output
function [z,dz,or] = fcn(q_dot,q)
% persistent dh_c
% if isempty(dh_c)
%     dh_c = Load_Franka_DH();
% end
[DH, Conv] = Load_Franka_DH();
z = zeros(3,1);
%z = get_pos(q);

[p,R] = DirectKinematic(DH,[q;0],Conv);
z = p;
phi = atan2(R(2,1),R(1,1));
teta = atan2(-R(3,1),sqrt(R(3,2)^2 + R(3,3)^2)); 
psi = atan2(R(3,2),R(3,3));
or = [phi teta psi]';

Ja = zeros(3,7);
Ja = get_Jacobianoa(q);

dz = zeros(3,1);
dz = Ja(1:3,1:7)*q_dot;

end

== matlab function franka_placement_task/PLANNER1/KZ_GENERATOR ==
  settings: updateMethod=DISCRETE  sampleTime=Ts
  data: k output; F_ext input; z input; z_des input; int input; comp input; e_max parameter; F_max parameter; F_int_max parameter
function k = fcn(F_ext, z, z_des, int, comp, e_max, F_max, F_int_max)
%% Description
% Set the K coefficient for a variable impedance controller based on a
% desired trajectory

%% Outputs
% k             stiffness

%% Inputs
% F_ext         measured external force
% z_des         desired trajectory
% z             current position
% int, comp     booleans for the interaction and compensation phase

%% Parameters
% F_int_max     desired interaction force
% F_max         nominal disturbance forces
% e_max         maximum steady-state error

%% persistent initialization
persistent ki kc F_comp int_prec comp_prec z_int z_int_dir 
if isempty(ki)
   ki = F_max/e_max;        % k obtained from interaction
end
if isempty(F_comp)
   F_comp = 0;              % weight to compensate
end
if isempty(kc)
      kc = F_max/e_max;     % k obtained from compensation
end
if isempty(z_int) 
    z_int = 1000;       % obstacle(or interaction) position
end
if isempty(z_int_dir) 
    z_int_dir = 0;          % prohibited direction due to the obstacle
end
if isempty(int_prec)
    int_prec = 0;           % previous values of int
end
if isempty(comp_prec)
    comp_prec = 0;          % previous values od comp
end

%% INTERACTION
% set ki in order to match a desired interaction force with the
% envirorment, and store interaction's position when detected
% X axes
if int == 1
    % detection of an interaction 
    if abs(F_ext-F_comp) > F_max
        if z_int == 1000                     % z_int has not been set yet
            z_int = z;
            z_int_dir = -sign(F_ext-F_comp);
        end
    end
    % setting of ki
    if abs(F_ext-F_comp) > F_int_max 
        % if interaction force is higher than threshold
        if ki*abs(z-z_des) > F_int_max
            ktemp_x = F_int_max/abs(z-z_des);
            if ktemp_x < ki                % ki needs to be only decreased
                ki = ktemp_x;
            end
        end
    end
end

%% COMPENSATION
% set kc in order to compensate the effect of the weight of the object,
% and store it
% X axes
if comp == 1
    % compensation detection
    if z_int == 1000                     % z_int not set before
       if abs(F_ext)/kc > e_max         
            kc = abs(F_ext)/e_max;
            F_comp = F_ext;
       end
    else 
        if z_int_dir == 1                % obstacle in above
            if z < z_int
                if abs(F_ext)/kc > e_max 
                    kc = abs(F_ext)/e_max;
                    F_comp = F_ext;
                end
            end
        else                                % obstacle is below
            if z > z_int
                if abs(F_ext)/kc > e_max
                    kc = abs(F_ext)/e_max;
                    F_comp = F_ext;
                end
            end
        end 
   end
end

%% reset to default values when comp or int shifts to zero
if comp==0 && comp_prec==1
    kc = F_max/e_max;
    F_comp = 0;
end
if int==0 && int_prec==1
    ki = F_max/e_max;
end

%% from int to comp and vice versa
if int==1 && int_prec==0
    if comp_prec == 1
        ki = kc;
    end
    z_int=1000;
    z_int_dir=0;
end
if comp == 1 && comp_prec==0
    if int_prec == 1
        kc = ki;
    end
end

% update to last booleans
int_prec = int;
comp_prec = comp;


%% Selection of Final Values of D-K
% default values
k = abs(F_max)/e_max;

% compensation
if comp == 1
    k = kc;
end

% both compensation and interaction are activated
% if "away" from obstacle set k = kc else ki
if int == 1
    k = ki;
    if comp == 1
        if z_int == 1000
            k = kc;                       % obstacle not reached
        else
            if z_int_dir == 1
                if z_des < z_int
                    k = kc;               % obstacle reached but "going away"
                end
            else
                if z_des > z_int
                    k = kc;               % obstacle reached but "going away"
                end
            end
        end
    else
        if z_int == 1000
            k = F_max/e_max;            % restore to default
        else
            if z_int_dir == 1
                if z_des < z_int
                    k = F_max/e_max;    % restore because "going away"
                end
            else
                if z_des > z_int
                    k = F_max/e_max;    % restore because "going away"
                end
            end
        end
    end
end

end

== matlab function franka_placement_task/direct kinematics1 ==
  data: q_dot input double; q input double; z output double; dz output double; or output
function [z,dz,or] = fcn(q_dot,q)
coder.extrinsic('get_Ja');
% persistent dh_c
% if isempty(dh_c)
%     dh_c = Load_Franka_DH();
% end
[DH, Conv] = Load_Franka_DH();
z = zeros(3,1);
%z = get_pos(q);

[p,R] = DirectKinematic(DH,[q;0],Conv);
z = p;
phi = atan2(R(2,1),R(1,1));
teta = atan2(-R(3,1),sqrt(R(3,2)^2 + R(3,3)^2)); 
psi = atan2(R(3,2),R(3,3));
or = [phi teta psi]';

Ja = zeros(6,7);
Ja = get_Ja(q);

dz = zeros(3,1);
dz = Ja(1:3,1:7)*q_dot;

end

== matlab function franka_placement_task/PLANNER/KD_INTERPOLATOR  ==
  settings: updateMethod=DISCRETE  sampleTime=Ts
  data: time input; K output; kx_f input; ky_f input; kz_f input; D output; e_max parameter; F_max parameter; M parameter; berta parameter; a0 parameter; mass parameter; csi parameter
function [K,D] = fcn(time, kx_f, ky_f, kz_f, e_max, F_max, M, berta, a0, mass, csi)
%% Description
% Interpolate K in order to guarantee stability

%% Outputs
% K             Stiffness matrix
% D             Damping matrix

%% Inputs
% kx_f, ky, f   desired values of K

%% Parameters
% F_max         nominal disturbance forces
% e_max         maximum steady-state error
% M             virtual mass
% berta, a0     parameters for the computation of stability conditions
% mass          virtual mass

%% persistent initialization
persistent kx ky kz time_prec
if isempty(time_prec)
    time_prec = 0;              % previous simulation time
end
if isempty(kx)
   kx = F_max/e_max;         % last value of k
end
if isempty(ky)
   ky = F_max/e_max;
end
if isempty(kz)
   kz = F_max/e_max;
end

% set k from desired one 
if kx_f <= kx       
    kx = kx_f;
else 
    % increese k in accordance with the stability conditions
    kx_i = kx;
    k_dotx = berta*(4*a0*sqrt(kx_i/mass)*(kx_i)^(3/2))/(sqrt(kx_i) + 2*a0*csi*sqrt(kx_i));
    k_tempx = kx_i + k_dotx*(time -time_prec);
    if k_tempx > kx_f
        kx = kx_f;
    else
        kx = k_tempx;
    end
end

% Y axes, same as X axes
if ky_f <= ky
    ky = ky_f;
else 
    ky_i = ky;
    k_doty = berta*(4*a0*sqrt(ky_i/mass)*(ky_i)^(3/2))/(sqrt(ky_i) + 2*a0*csi*sqrt(ky_i));
    k_tempy = ky_i + k_doty*(time -time_prec);
    if k_tempy > ky_f
        ky = ky_f;
    else
        ky = k_tempy;
    end
end

% Z axes, same as other axes
if kz_f <= kz
    kz = kz_f;
else 
    kz_i = kz;
    k_dotz = berta*(4*a0*sqrt(kz_i/mass)*(kz_i)^(3/2))/(sqrt(kz_i) + 2*a0*csi*sqrt(kz_i));
    k_tempz = kz_i + k_dotz*(time -time_prec);
    if k_tempz > kz_f
        kz = kz_f;
    else
        kz = k_tempz;
    end
end

time_prec = time;

% damping computation, critically damped condition
dx = sqrt(4*kx*M);
dy = sqrt(4*ky*M);
dz = sqrt(4*kz*M);

%% Final impedance matrices
D = diag([dx, dy, dz]);
K = diag([kx, ky, kz]);

end

== matlab function franka_placement_task/PLANNER/KX_GENERATOR ==
  settings: updateMethod=DISCRETE  sampleTime=Ts
  data: k output; F_ext input; z input; z_des input; int input; comp input; e_max parameter; F_max parameter; F_int_max parameter
function k = fcn(F_ext, z, z_des, int, comp, e_max, F_max, F_int_max)
%% Description
% Set the K coefficient for a variable impedance controller based on a
% desired trajectory

%% Outputs
% k             stiffness

%% Inputs
% F_ext         measured external force
% z_des         desired trajectory
% z             current position
% int, comp     booleans for the interaction and compensation phase

%% Parameters
% F_int_max     desired interaction force
% F_max         nominal disturbance forces
% e_max         maximum steady-state error

%% persistent initialization
persistent ki kc F_comp int_prec comp_prec z_int z_int_dir 
if isempty(ki)
   ki = F_max/e_max;        % k obtained from interaction
end
if isempty(F_comp)
   F_comp = 0;              % weight to compensate
end
if isempty(kc)
      kc = F_max/e_max;     % k obtained from compensation
end
if isempty(z_int) 
    z_int = 1000;       % obstacle(or interaction) position
end
if isempty(z_int_dir) 
    z_int_dir = 0;          % prohibited direction due to the obstacle
end
if isempty(int_prec)
    int_prec = 0;           % previous values of int
end
if isempty(comp_prec)
    comp_prec = 0;          % previous values od comp
end

%% INTERACTION
% set ki in order to match a desired interaction force with the
% envirorment, and store interaction's position when detected
% X axes
if int == 1
    % detection of an interaction 
    if abs(F_ext-F_comp) > F_max
        if z_int == 1000                     % z_int has not been set yet
            z_int = z;
            z_int_dir = -sign(F_ext-F_comp);
        end
    end
    % setting of ki
    if abs(F_ext-F_comp) > F_int_max 
        % if interaction force is higher than threshold
        if ki*abs(z-z_des) > F_int_max
            ktemp_x = F_int_max/abs(z-z_des);
            if ktemp_x < ki                % ki needs to be only decreased
                ki = ktemp_x;
            end
        end
    end
end

%% COMPENSATION
% set kc in order to compensate the effect of the weight of the object,
% and store it
% X axes
if comp == 1
    % compensation detection
    if z_int == 1000                     % z_int not set before
       if abs(F_ext)/kc > e_max         
            kc = abs(F_ext)/e_max;
            F_comp = F_ext;
       end
    else 
        if z_int_dir == 1                % obstacle in above
            if z < z_int
                if abs(F_ext)/kc > e_max 
                    kc = abs(F_ext)/e_max;
                    F_comp = F_ext;
                end
            end
        else                                % obstacle is below
            if z > z_int
                if abs(F_ext)/kc > e_max
                    kc = abs(F_ext)/e_max;
                    F_comp = F_ext;
                end
            end
        end 
   end
end

%% reset to default values when comp or int shifts to zero
if comp==0 && comp_prec==1
    kc = F_max/e_max;
    F_comp = 0;
end
if int==0 && int_prec==1
    ki = F_max/e_max;
end

%% from int to comp and vice versa
if int==1 && int_prec==0
    if comp_prec == 1
        ki = kc;
    end
    z_int=1000;
    z_int_dir=0;
end
if comp == 1 && comp_prec==0
    if int_prec == 1
        kc = ki;
    end
end

% update to last booleans
int_prec = int;
comp_prec = comp;


%% Selection of Final Values of D-K
% default values
k = abs(F_max)/e_max;

% compensation
if comp == 1
    k = kc;
end

% both compensation and interaction are activated
% if "away" from obstacle set k = kc else ki
if int == 1
    k = ki;
    if comp == 1
        if z_int == 1000
            k = kc;                       % obstacle not reached
        else
            if z_int_dir == 1
                if z_des < z_int
                    k = kc;               % obstacle reached but "going away"
                end
            else
                if z_des > z_int
                    k = kc;               % obstacle reached but "going away"
                end
            end
        end
    else
        if z_int == 1000
            k = F_max/e_max;            % restore to default
        else
            if z_int_dir == 1
                if z_des < z_int
                    k = F_max/e_max;    % restore because "going away"
                end
            else
                if z_des > z_int
                    k = F_max/e_max;    % restore because "going away"
                end
            end
        end
    end
end

end

== matlab function franka_placement_task/TRAJECTORY/INTERPOLATOR ==
  data: xi input; z_des output; xf input; tf input; t input; v input; alpha input; dz_des output; ddz_des output
function [z_des, dz_des, ddz_des] = fcn(xi, xf, tf, t, v, alpha)

ta = alpha*tf; 
xa = (1/2)*v*ta;

if t >= 0 && t < ta
    ddz_des = v./ta;
    dz_des = ddz_des*t;
    z_des = xi + (1/2)*ddz_des*t^2;
elseif t >= ta && t < (tf-ta)
    ddz_des = [0; 0; 0]; 
    dz_des = v; 
    z_des = xi + xa + dz_des*(t-ta);
elseif t >= (tf- ta) && t < tf
    ddz_des = -v./ta;
    dz_des = v + ddz_des*(t - (tf-ta));
    z_des = xi + xa + v*(tf-2*ta) + v*(t-(tf-ta)) + (1/2)*ddz_des*(t-(tf-ta))^2;
else 
    ddz_des = [0; 0; 0];
    dz_des = [0; 0; 0];
    z_des = xf;
end

end
